simulink model "Assignment_3"  (R2020b)
settings: Solver=VariableStepAuto  StartTime=0.0  StopTime=10.0  RelTol=1e-3
settings Model: Creator=Shantam Garg  LastModifiedBy=Shantam Garg

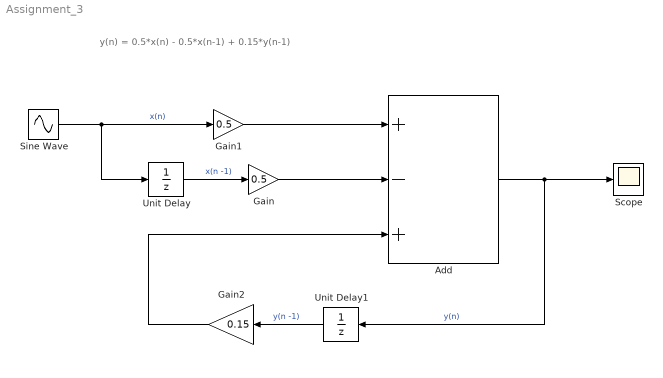
== system Assignment_3 ==
  note: y(n) = 0.5*x(n) - 0.5*x(n-1) + 0.15*y(n-1)
  Add : Sum  Inputs=+-+
  Gain : Gain  Gain=0.5
  Gain1 : Gain  Gain=0.5
  Gain2 : Gain  Gain=0.15
  Scope : Scope
  Sine Wave : Sin  Frequency=1000  SampleTime=0
  Unit Delay : UnitDelay  SampleTime=-1  HasFrameUpgradeWarning=on
  Unit Delay1 : UnitDelay  SampleTime=-1  HasFrameUpgradeWarning=on
  wires:
  Sine Wave/1 -> Unit Delay/1, Gain1/1  "x(n)"
  Unit Delay/1 -> Gain/1  "x(n -1)"
  Gain1/1 -> Add/1
  Gain/1 -> Add/2
  Add/1 -> Scope/1, Unit Delay1/1  "y(n)"
  Unit Delay1/1 -> Gain2/1  "y(n -1)"
  Gain2/1 -> Add/3
